simulink model "DC_response"  (R2020b)
settings: Solver=VariableStepAuto  StartTime=0.0  StopTime=10.0  RelTol=1e-3
model workspace: external: MATLAB File C:\Users\deves\MATLAB\Projects\problem5\data5.m (data not in the file)
values from neighbouring files (symbols this model uses):
  C = 10    [data5.m]
  R = 10    [data5.m]
settings Model: Creator=deves  LastModifiedBy=deves

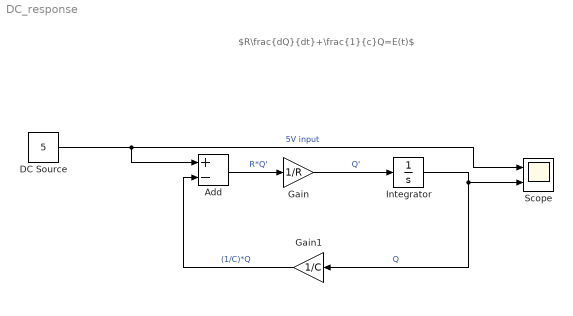
== system DC_response ==
  note: $R\frac{dQ}{dt}+\frac{1}{c}Q=E(t)$
  Add : Sum  Inputs=+-
  DC Source : Constant  Value=5
  Gain : Gain  Gain=1/R
  Gain1 : Gain  Gain=1/C
  Integrator : Integrator  InitialCondition=-1
  Scope : Scope  NumInputPorts=2
  wires:
  Integrator/1 -> Gain1/1, Scope/2  "Q"
  DC Source/1 -> Scope/1, Add/1  "5V input"
  Gain/1 -> Integrator/1  "Q'"
  Gain1/1 -> Add/2  "(1/C)*Q"
  Add/1 -> Gain/1  "R*Q'"
